simulink model "cpu2"  (R2020a)
settings: Solver=VariableStepAuto  StartTime=0.0  StopTime=10.0  RelTol=1e-3
libraries: simulink_extras x402, msbPllFoundation x1
(part 25 of 63)

== system cpu2/ALU/Multiplier/Subsystem2/Subsystem1/Subsystem1/Subsystem12 ==
  In1 : Inport
  In2 : Inport  Port=2
  Logical Operator1 : Logic  Operator=XOR  AllPortsSameDT=off  OutDataTypeStr=boolean
  Logical Operator2 : Logic  AllPortsSameDT=off  OutDataTypeStr=boolean
  Out1 : Outport
  Out2 : Outport  Port=2
  wires:
  In1/1 -> Logical Operator2/1, Logical Operator1/1
  Logical Operator1/1 -> Out1/1
  Logical Operator2/1 -> Out2/1
  In2/1 -> Logical Operator1/2, Logical Operator2/2

== system cpu2/ALU/Multiplier/Subsystem2/Subsystem1/Subsystem1/Subsystem13 ==
  In1 : Inport
  In2 : Inport  Port=2
  Logical Operator1 : Logic  Operator=XOR  AllPortsSameDT=off  OutDataTypeStr=boolean
  Logical Operator2 : Logic  AllPortsSameDT=off  OutDataTypeStr=boolean
  Out1 : Outport
  Out2 : Outport  Port=2
  wires:
  In1/1 -> Logical Operator2/1, Logical Operator1/1
  Logical Operator1/1 -> Out1/1
  Logical Operator2/1 -> Out2/1
  In2/1 -> Logical Operator1/2, Logical Operator2/2

== system cpu2/ALU/Multiplier/Subsystem2/Subsystem1/Subsystem1/Subsystem14 ==
  In1 : Inport
  In2 : Inport  Port=2
  Logical Operator1 : Logic  Operator=XOR  AllPortsSameDT=off  OutDataTypeStr=boolean
  Logical Operator2 : Logic  AllPortsSameDT=off  OutDataTypeStr=boolean
  Out1 : Outport
  Out2 : Outport  Port=2
  wires:
  In1/1 -> Logical Operator2/1, Logical Operator1/1
  Logical Operator1/1 -> Out1/1
  Logical Operator2/1 -> Out2/1
  In2/1 -> Logical Operator1/2, Logical Operator2/2

== system cpu2/ALU/Multiplier/Subsystem2/Subsystem1/Subsystem1/Subsystem2 ==
  In1 : Inport
  In2 : Inport  Port=2
  Logical Operator1 : Logic  Operator=XOR  AllPortsSameDT=off  OutDataTypeStr=boolean
  Logical Operator2 : Logic  AllPortsSameDT=off  OutDataTypeStr=boolean
  Out1 : Outport
  Out2 : Outport  Port=2
  wires:
  In1/1 -> Logical Operator2/1, Logical Operator1/1
  Logical Operator1/1 -> Out1/1
  Logical Operator2/1 -> Out2/1
  In2/1 -> Logical Operator1/2, Logical Operator2/2

== system cpu2/ALU/Multiplier/Subsystem2/Subsystem1/Subsystem1/Subsystem3 ==
  In1 : Inport
  In2 : Inport  Port=2
  In3 : Inport  Port=3
  Logical Operator : Logic  Operator=XOR  AllPortsSameDT=off  OutDataTypeStr=boolean
  Logical Operator1 : Logic  Operator=XOR  AllPortsSameDT=off  OutDataTypeStr=boolean
  Logical Operator2 : Logic  AllPortsSameDT=off  OutDataTypeStr=boolean
  Logical Operator3 : Logic  AllPortsSameDT=off  OutDataTypeStr=boolean
  Logical Operator4 : Logic  Operator=OR  AllPortsSameDT=off  OutDataTypeStr=boolean
  Out1 : Outport
  Out2 : Outport  Port=2
  wires:
  Logical Operator1/1 -> Out1/1
  Logical Operator2/1 -> Logical Operator4/1
  Logical Operator4/1 -> Out2/1
  In3/1 -> Logical Operator2/2, Logical Operator1/2
  In2/1 -> Logical Operator3/2, Logical Operator/2
  In1/1 -> Logical Operator3/1, Logical Operator/1
  Logical Operator3/1 -> Logical Operator4/2
  Logical Operator/1 -> Logical Operator2/1, Logical Operator1/1

== system cpu2/ALU/Multiplier/Subsystem2/Subsystem1/Subsystem1/Subsystem4 ==
  In1 : Inport
  In2 : Inport  Port=2
  In3 : Inport  Port=3
  Logical Operator : Logic  Operator=XOR  AllPortsSameDT=off  OutDataTypeStr=boolean
  Logical Operator1 : Logic  Operator=XOR  AllPortsSameDT=off  OutDataTypeStr=boolean
  Logical Operator2 : Logic  AllPortsSameDT=off  OutDataTypeStr=boolean
  Logical Operator3 : Logic  AllPortsSameDT=off  OutDataTypeStr=boolean
  Logical Operator4 : Logic  Operator=OR  AllPortsSameDT=off  OutDataTypeStr=boolean
  Out1 : Outport
  Out2 : Outport  Port=2
  wires:
  Logical Operator1/1 -> Out1/1
  Logical Operator2/1 -> Logical Operator4/1
  Logical Operator4/1 -> Out2/1
  In3/1 -> Logical Operator2/2, Logical Operator1/2
  In2/1 -> Logical Operator3/2, Logical Operator/2
  In1/1 -> Logical Operator3/1, Logical Operator/1
  Logical Operator3/1 -> Logical Operator4/2
  Logical Operator/1 -> Logical Operator2/1, Logical Operator1/1

== system cpu2/ALU/Multiplier/Subsystem2/Subsystem1/Subsystem1/Subsystem5 ==
  In1 : Inport
  In2 : Inport  Port=2
  Logical Operator1 : Logic  Operator=XOR  AllPortsSameDT=off  OutDataTypeStr=boolean
  Logical Operator2 : Logic  AllPortsSameDT=off  OutDataTypeStr=boolean
  Out1 : Outport
  Out2 : Outport  Port=2
  wires:
  In1/1 -> Logical Operator2/1, Logical Operator1/1
  Logical Operator1/1 -> Out1/1
  Logical Operator2/1 -> Out2/1
  In2/1 -> Logical Operator1/2, Logical Operator2/2

== system cpu2/ALU/Multiplier/Subsystem2/Subsystem1/Subsystem1/Subsystem6 ==
  In1 : Inport
  In2 : Inport  Port=2
  In3 : Inport  Port=3
  Logical Operator : Logic  Operator=XOR  AllPortsSameDT=off  OutDataTypeStr=boolean
  Logical Operator1 : Logic  Operator=XOR  AllPortsSameDT=off  OutDataTypeStr=boolean
  Logical Operator2 : Logic  AllPortsSameDT=off  OutDataTypeStr=boolean
  Logical Operator3 : Logic  AllPortsSameDT=off  OutDataTypeStr=boolean
  Logical Operator4 : Logic  Operator=OR  AllPortsSameDT=off  OutDataTypeStr=boolean
  Out1 : Outport
  Out2 : Outport  Port=2
  wires:
  Logical Operator1/1 -> Out1/1
  Logical Operator2/1 -> Logical Operator4/1
  Logical Operator4/1 -> Out2/1
  In3/1 -> Logical Operator2/2, Logical Operator1/2
  In2/1 -> Logical Operator3/2, Logical Operator/2
  In1/1 -> Logical Operator3/1, Logical Operator/1
  Logical Operator3/1 -> Logical Operator4/2
  Logical Operator/1 -> Logical Operator2/1, Logical Operator1/1

== system cpu2/ALU/Multiplier/Subsystem2/Subsystem1/Subsystem1/Subsystem7 ==
  In1 : Inport
  In2 : Inport  Port=2
  In3 : Inport  Port=3
  Logical Operator : Logic  Operator=XOR  AllPortsSameDT=off  OutDataTypeStr=boolean
  Logical Operator1 : Logic  Operator=XOR  AllPortsSameDT=off  OutDataTypeStr=boolean
  Logical Operator2 : Logic  AllPortsSameDT=off  OutDataTypeStr=boolean
  Logical Operator3 : Logic  AllPortsSameDT=off  OutDataTypeStr=boolean
  Logical Operator4 : Logic  Operator=OR  AllPortsSameDT=off  OutDataTypeStr=boolean
  Out1 : Outport
  Out2 : Outport  Port=2
  wires:
  Logical Operator1/1 -> Out1/1
  Logical Operator2/1 -> Logical Operator4/1
  Logical Operator4/1 -> Out2/1
  In3/1 -> Logical Operator2/2, Logical Operator1/2
  In2/1 -> Logical Operator3/2, Logical Operator/2
  In1/1 -> Logical Operator3/1, Logical Operator/1
  Logical Operator3/1 -> Logical Operator4/2
  Logical Operator/1 -> Logical Operator2/1, Logical Operator1/1

== system cpu2/ALU/Multiplier/Subsystem2/Subsystem1/Subsystem1/Subsystem8 ==
  In1 : Inport
  In2 : Inport  Port=2
  In3 : Inport  Port=3
  Logical Operator : Logic  Operator=XOR  AllPortsSameDT=off  OutDataTypeStr=boolean
  Logical Operator1 : Logic  Operator=XOR  AllPortsSameDT=off  OutDataTypeStr=boolean
  Logical Operator2 : Logic  AllPortsSameDT=off  OutDataTypeStr=boolean
  Logical Operator3 : Logic  AllPortsSameDT=off  OutDataTypeStr=boolean
  Logical Operator4 : Logic  Operator=OR  AllPortsSameDT=off  OutDataTypeStr=boolean
  Out1 : Outport
  Out2 : Outport  Port=2
  wires:
  Logical Operator1/1 -> Out1/1
  Logical Operator2/1 -> Logical Operator4/1
  Logical Operator4/1 -> Out2/1
  In3/1 -> Logical Operator2/2, Logical Operator1/2
  In2/1 -> Logical Operator3/2, Logical Operator/2
  In1/1 -> Logical Operator3/1, Logical Operator/1
  Logical Operator3/1 -> Logical Operator4/2
  Logical Operator/1 -> Logical Operator2/1, Logical Operator1/1

== system cpu2/ALU/Multiplier/Subsystem2/Subsystem1/Subsystem1/Subsystem9 ==
  In1 : Inport
  In2 : Inport  Port=2
  In3 : Inport  Port=3
  Logical Operator : Logic  Operator=XOR  AllPortsSameDT=off  OutDataTypeStr=boolean
  Logical Operator1 : Logic  Operator=XOR  AllPortsSameDT=off  OutDataTypeStr=boolean
  Logical Operator2 : Logic  AllPortsSameDT=off  OutDataTypeStr=boolean
  Logical Operator3 : Logic  AllPortsSameDT=off  OutDataTypeStr=boolean
  Logical Operator4 : Logic  Operator=OR  AllPortsSameDT=off  OutDataTypeStr=boolean
  Out1 : Outport
  Out2 : Outport  Port=2
  wires:
  Logical Operator1/1 -> Out1/1
  Logical Operator2/1 -> Logical Operator4/1
  Logical Operator4/1 -> Out2/1
  In3/1 -> Logical Operator2/2, Logical Operator1/2
  In2/1 -> Logical Operator3/2, Logical Operator/2
  In1/1 -> Logical Operator3/1, Logical Operator/1
  Logical Operator3/1 -> Logical Operator4/2
  Logical Operator/1 -> Logical Operator2/1, Logical Operator1/1

== system cpu2/ALU/Multiplier/Subsystem2/Subsystem1/Subsystem15/Subsystem ==
  In1 : Inport
  In2 : Inport  Port=2
  Logical Operator1 : Logic  Operator=XOR  AllPortsSameDT=off  OutDataTypeStr=boolean
  Logical Operator2 : Logic  AllPortsSameDT=off  OutDataTypeStr=boolean
  Out1 : Outport
  Out2 : Outport  Port=2
  wires:
  In1/1 -> Logical Operator2/1, Logical Operator1/1
  Logical Operator1/1 -> Out1/1
  Logical Operator2/1 -> Out2/1
  In2/1 -> Logical Operator1/2, Logical Operator2/2

== system cpu2/ALU/Multiplier/Subsystem2/Subsystem1/Subsystem15/Subsystem1 ==
  In1 : Inport
  In2 : Inport  Port=2
  In3 : Inport  Port=3
  Logical Operator : Logic  Operator=XOR  AllPortsSameDT=off  OutDataTypeStr=boolean
  Logical Operator1 : Logic  Operator=XOR  AllPortsSameDT=off  OutDataTypeStr=boolean
  Logical Operator2 : Logic  AllPortsSameDT=off  OutDataTypeStr=boolean
  Logical Operator3 : Logic  AllPortsSameDT=off  OutDataTypeStr=boolean
  Logical Operator4 : Logic  Operator=OR  AllPortsSameDT=off  OutDataTypeStr=boolean
  Out1 : Outport
  Out2 : Outport  Port=2
  wires:
  Logical Operator1/1 -> Out1/1
  Logical Operator2/1 -> Logical Operator4/1
  Logical Operator4/1 -> Out2/1
  In3/1 -> Logical Operator2/2, Logical Operator1/2
  In2/1 -> Logical Operator3/2, Logical Operator/2
  In1/1 -> Logical Operator3/1, Logical Operator/1
  Logical Operator3/1 -> Logical Operator4/2
  Logical Operator/1 -> Logical Operator2/1, Logical Operator1/1

== system cpu2/ALU/Multiplier/Subsystem2/Subsystem1/Subsystem15/Subsystem10 ==
  In1 : Inport
  In2 : Inport  Port=2
  Logical Operator1 : Logic  Operator=XOR  AllPortsSameDT=off  OutDataTypeStr=boolean
  Logical Operator2 : Logic  AllPortsSameDT=off  OutDataTypeStr=boolean
  Out1 : Outport
  Out2 : Outport  Port=2
  wires:
  In1/1 -> Logical Operator2/1, Logical Operator1/1
  Logical Operator1/1 -> Out1/1
  Logical Operator2/1 -> Out2/1
  In2/1 -> Logical Operator1/2, Logical Operator2/2

== system cpu2/ALU/Multiplier/Subsystem2/Subsystem1/Subsystem15/Subsystem11 ==
  In1 : Inport
  In2 : Inport  Port=2
  Logical Operator1 : Logic  Operator=XOR  AllPortsSameDT=off  OutDataTypeStr=boolean
  Logical Operator2 : Logic  AllPortsSameDT=off  OutDataTypeStr=boolean
  Out1 : Outport
  Out2 : Outport  Port=2
  wires:
  In1/1 -> Logical Operator2/1, Logical Operator1/1
  Logical Operator1/1 -> Out1/1
  Logical Operator2/1 -> Out2/1
  In2/1 -> Logical Operator1/2, Logical Operator2/2

== system cpu2/ALU/Multiplier/Subsystem2/Subsystem1/Subsystem15/Subsystem12 ==
  In1 : Inport
  In2 : Inport  Port=2
  Logical Operator1 : Logic  Operator=XOR  AllPortsSameDT=off  OutDataTypeStr=boolean
  Logical Operator2 : Logic  AllPortsSameDT=off  OutDataTypeStr=boolean
  Out1 : Outport
  Out2 : Outport  Port=2
  wires:
  In1/1 -> Logical Operator2/1, Logical Operator1/1
  Logical Operator1/1 -> Out1/1
  Logical Operator2/1 -> Out2/1
  In2/1 -> Logical Operator1/2, Logical Operator2/2

== system cpu2/ALU/Multiplier/Subsystem2/Subsystem1/Subsystem15/Subsystem13 ==
  In1 : Inport
  In2 : Inport  Port=2
  Logical Operator1 : Logic  Operator=XOR  AllPortsSameDT=off  OutDataTypeStr=boolean
  Logical Operator2 : Logic  AllPortsSameDT=off  OutDataTypeStr=boolean
  Out1 : Outport
  Out2 : Outport  Port=2
  wires:
  In1/1 -> Logical Operator2/1, Logical Operator1/1
  Logical Operator1/1 -> Out1/1
  Logical Operator2/1 -> Out2/1
  In2/1 -> Logical Operator1/2, Logical Operator2/2

== system cpu2/ALU/Multiplier/Subsystem2/Subsystem1/Subsystem15/Subsystem14 ==
  In1 : Inport
  In2 : Inport  Port=2
  Logical Operator1 : Logic  Operator=XOR  AllPortsSameDT=off  OutDataTypeStr=boolean
  Logical Operator2 : Logic  AllPortsSameDT=off  OutDataTypeStr=boolean
  Out1 : Outport
  Out2 : Outport  Port=2
  wires:
  In1/1 -> Logical Operator2/1, Logical Operator1/1
  Logical Operator1/1 -> Out1/1
  Logical Operator2/1 -> Out2/1
  In2/1 -> Logical Operator1/2, Logical Operator2/2

== system cpu2/ALU/Multiplier/Subsystem2/Subsystem1/Subsystem15/Subsystem2 ==
  In1 : Inport
  In2 : Inport  Port=2
  Logical Operator1 : Logic  Operator=XOR  AllPortsSameDT=off  OutDataTypeStr=boolean
  Logical Operator2 : Logic  AllPortsSameDT=off  OutDataTypeStr=boolean
  Out1 : Outport
  Out2 : Outport  Port=2
  wires:
  In1/1 -> Logical Operator2/1, Logical Operator1/1
  Logical Operator1/1 -> Out1/1
  Logical Operator2/1 -> Out2/1
  In2/1 -> Logical Operator1/2, Logical Operator2/2

== system cpu2/ALU/Multiplier/Subsystem2/Subsystem1/Subsystem15/Subsystem3 ==
  In1 : Inport
  In2 : Inport  Port=2
  In3 : Inport  Port=3
  Logical Operator : Logic  Operator=XOR  AllPortsSameDT=off  OutDataTypeStr=boolean
  Logical Operator1 : Logic  Operator=XOR  AllPortsSameDT=off  OutDataTypeStr=boolean
  Logical Operator2 : Logic  AllPortsSameDT=off  OutDataTypeStr=boolean
  Logical Operator3 : Logic  AllPortsSameDT=off  OutDataTypeStr=boolean
  Logical Operator4 : Logic  Operator=OR  AllPortsSameDT=off  OutDataTypeStr=boolean
  Out1 : Outport
  Out2 : Outport  Port=2
  wires:
  Logical Operator1/1 -> Out1/1
  Logical Operator2/1 -> Logical Operator4/1
  Logical Operator4/1 -> Out2/1
  In3/1 -> Logical Operator2/2, Logical Operator1/2
  In2/1 -> Logical Operator3/2, Logical Operator/2
  In1/1 -> Logical Operator3/1, Logical Operator/1
  Logical Operator3/1 -> Logical Operator4/2
  Logical Operator/1 -> Logical Operator2/1, Logical Operator1/1

== system cpu2/ALU/Multiplier/Subsystem2/Subsystem1/Subsystem15/Subsystem4 ==
  In1 : Inport
  In2 : Inport  Port=2
  In3 : Inport  Port=3
  Logical Operator : Logic  Operator=XOR  AllPortsSameDT=off  OutDataTypeStr=boolean
  Logical Operator1 : Logic  Operator=XOR  AllPortsSameDT=off  OutDataTypeStr=boolean
  Logical Operator2 : Logic  AllPortsSameDT=off  OutDataTypeStr=boolean
  Logical Operator3 : Logic  AllPortsSameDT=off  OutDataTypeStr=boolean
  Logical Operator4 : Logic  Operator=OR  AllPortsSameDT=off  OutDataTypeStr=boolean
  Out1 : Outport
  Out2 : Outport  Port=2
  wires:
  Logical Operator1/1 -> Out1/1
  Logical Operator2/1 -> Logical Operator4/1
  Logical Operator4/1 -> Out2/1
  In3/1 -> Logical Operator2/2, Logical Operator1/2
  In2/1 -> Logical Operator3/2, Logical Operator/2
  In1/1 -> Logical Operator3/1, Logical Operator/1
  Logical Operator3/1 -> Logical Operator4/2
  Logical Operator/1 -> Logical Operator2/1, Logical Operator1/1

== system cpu2/ALU/Multiplier/Subsystem2/Subsystem1/Subsystem15/Subsystem5 ==
  In1 : Inport
  In2 : Inport  Port=2
  Logical Operator1 : Logic  Operator=XOR  AllPortsSameDT=off  OutDataTypeStr=boolean
  Logical Operator2 : Logic  AllPortsSameDT=off  OutDataTypeStr=boolean
  Out1 : Outport
  Out2 : Outport  Port=2
  wires:
  In1/1 -> Logical Operator2/1, Logical Operator1/1
  Logical Operator1/1 -> Out1/1
  Logical Operator2/1 -> Out2/1
  In2/1 -> Logical Operator1/2, Logical Operator2/2

== system cpu2/ALU/Multiplier/Subsystem2/Subsystem1/Subsystem15/Subsystem6 ==
  In1 : Inport
  In2 : Inport  Port=2
  In3 : Inport  Port=3
  Logical Operator : Logic  Operator=XOR  AllPortsSameDT=off  OutDataTypeStr=boolean
  Logical Operator1 : Logic  Operator=XOR  AllPortsSameDT=off  OutDataTypeStr=boolean
  Logical Operator2 : Logic  AllPortsSameDT=off  OutDataTypeStr=boolean
  Logical Operator3 : Logic  AllPortsSameDT=off  OutDataTypeStr=boolean
  Logical Operator4 : Logic  Operator=OR  AllPortsSameDT=off  OutDataTypeStr=boolean
  Out1 : Outport
  Out2 : Outport  Port=2
  wires:
  Logical Operator1/1 -> Out1/1
  Logical Operator2/1 -> Logical Operator4/1
  Logical Operator4/1 -> Out2/1
  In3/1 -> Logical Operator2/2, Logical Operator1/2
  In2/1 -> Logical Operator3/2, Logical Operator/2
  In1/1 -> Logical Operator3/1, Logical Operator/1
  Logical Operator3/1 -> Logical Operator4/2
  Logical Operator/1 -> Logical Operator2/1, Logical Operator1/1

== system cpu2/ALU/Multiplier/Subsystem2/Subsystem1/Subsystem15/Subsystem7 ==
  In1 : Inport
  In2 : Inport  Port=2
  In3 : Inport  Port=3
  Logical Operator : Logic  Operator=XOR  AllPortsSameDT=off  OutDataTypeStr=boolean
  Logical Operator1 : Logic  Operator=XOR  AllPortsSameDT=off  OutDataTypeStr=boolean
  Logical Operator2 : Logic  AllPortsSameDT=off  OutDataTypeStr=boolean
  Logical Operator3 : Logic  AllPortsSameDT=off  OutDataTypeStr=boolean
  Logical Operator4 : Logic  Operator=OR  AllPortsSameDT=off  OutDataTypeStr=boolean
  Out1 : Outport
  Out2 : Outport  Port=2
  wires:
  Logical Operator1/1 -> Out1/1
  Logical Operator2/1 -> Logical Operator4/1
  Logical Operator4/1 -> Out2/1
  In3/1 -> Logical Operator2/2, Logical Operator1/2
  In2/1 -> Logical Operator3/2, Logical Operator/2
  In1/1 -> Logical Operator3/1, Logical Operator/1
  Logical Operator3/1 -> Logical Operator4/2
  Logical Operator/1 -> Logical Operator2/1, Logical Operator1/1

== system cpu2/ALU/Multiplier/Subsystem2/Subsystem1/Subsystem15/Subsystem8 ==
  In1 : Inport
  In2 : Inport  Port=2
  In3 : Inport  Port=3
  Logical Operator : Logic  Operator=XOR  AllPortsSameDT=off  OutDataTypeStr=boolean
  Logical Operator1 : Logic  Operator=XOR  AllPortsSameDT=off  OutDataTypeStr=boolean
  Logical Operator2 : Logic  AllPortsSameDT=off  OutDataTypeStr=boolean
  Logical Operator3 : Logic  AllPortsSameDT=off  OutDataTypeStr=boolean
  Logical Operator4 : Logic  Operator=OR  AllPortsSameDT=off  OutDataTypeStr=boolean
  Out1 : Outport
  Out2 : Outport  Port=2
  wires:
  Logical Operator1/1 -> Out1/1
  Logical Operator2/1 -> Logical Operator4/1
  Logical Operator4/1 -> Out2/1
  In3/1 -> Logical Operator2/2, Logical Operator1/2
  In2/1 -> Logical Operator3/2, Logical Operator/2
  In1/1 -> Logical Operator3/1, Logical Operator/1
  Logical Operator3/1 -> Logical Operator4/2
  Logical Operator/1 -> Logical Operator2/1, Logical Operator1/1

== system cpu2/ALU/Multiplier/Subsystem2/Subsystem1/Subsystem15/Subsystem9 ==
  In1 : Inport
  In2 : Inport  Port=2
  In3 : Inport  Port=3
  Logical Operator : Logic  Operator=XOR  AllPortsSameDT=off  OutDataTypeStr=boolean
  Logical Operator1 : Logic  Operator=XOR  AllPortsSameDT=off  OutDataTypeStr=boolean
  Logical Operator2 : Logic  AllPortsSameDT=off  OutDataTypeStr=boolean
  Logical Operator3 : Logic  AllPortsSameDT=off  OutDataTypeStr=boolean
  Logical Operator4 : Logic  Operator=OR  AllPortsSameDT=off  OutDataTypeStr=boolean
  Out1 : Outport
  Out2 : Outport  Port=2
  wires:
  Logical Operator1/1 -> Out1/1
  Logical Operator2/1 -> Logical Operator4/1
  Logical Operator4/1 -> Out2/1
  In3/1 -> Logical Operator2/2, Logical Operator1/2
  In2/1 -> Logical Operator3/2, Logical Operator/2
  In1/1 -> Logical Operator3/1, Logical Operator/1
  Logical Operator3/1 -> Logical Operator4/2
  Logical Operator/1 -> Logical Operator2/1, Logical Operator1/1

== system cpu2/ALU/Multiplier/Subsystem2/Subsystem1/Subsystem2/Subsystem ==
  In1 : Inport
  In2 : Inport  Port=2
  Logical Operator1 : Logic  Operator=XOR  AllPortsSameDT=off  OutDataTypeStr=boolean
  Logical Operator2 : Logic  AllPortsSameDT=off  OutDataTypeStr=boolean
  Out1 : Outport
  Out2 : Outport  Port=2
  wires:
  In1/1 -> Logical Operator2/1, Logical Operator1/1
  Logical Operator1/1 -> Out1/1
  Logical Operator2/1 -> Out2/1
  In2/1 -> Logical Operator1/2, Logical Operator2/2

== system cpu2/ALU/Multiplier/Subsystem2/Subsystem1/Subsystem2/Subsystem1 ==
  In1 : Inport
  In2 : Inport  Port=2
  In3 : Inport  Port=3
  Logical Operator : Logic  Operator=XOR  AllPortsSameDT=off  OutDataTypeStr=boolean
  Logical Operator1 : Logic  Operator=XOR  AllPortsSameDT=off  OutDataTypeStr=boolean
  Logical Operator2 : Logic  AllPortsSameDT=off  OutDataTypeStr=boolean
  Logical Operator3 : Logic  AllPortsSameDT=off  OutDataTypeStr=boolean
  Logical Operator4 : Logic  Operator=OR  AllPortsSameDT=off  OutDataTypeStr=boolean
  Out1 : Outport
  Out2 : Outport  Port=2
  wires:
  Logical Operator1/1 -> Out1/1
  Logical Operator2/1 -> Logical Operator4/1
  Logical Operator4/1 -> Out2/1
  In3/1 -> Logical Operator2/2, Logical Operator1/2
  In2/1 -> Logical Operator3/2, Logical Operator/2
  In1/1 -> Logical Operator3/1, Logical Operator/1
  Logical Operator3/1 -> Logical Operator4/2
  Logical Operator/1 -> Logical Operator2/1, Logical Operator1/1

== system cpu2/ALU/Multiplier/Subsystem2/Subsystem1/Subsystem2/Subsystem10 ==
  In1 : Inport
  In2 : Inport  Port=2
  Logical Operator1 : Logic  Operator=XOR  AllPortsSameDT=off  OutDataTypeStr=boolean
  Logical Operator2 : Logic  AllPortsSameDT=off  OutDataTypeStr=boolean
  Out1 : Outport
  Out2 : Outport  Port=2
  wires:
  In1/1 -> Logical Operator2/1, Logical Operator1/1
  Logical Operator1/1 -> Out1/1
  Logical Operator2/1 -> Out2/1
  In2/1 -> Logical Operator1/2, Logical Operator2/2

== system cpu2/ALU/Multiplier/Subsystem2/Subsystem1/Subsystem2/Subsystem11 ==
  In1 : Inport
  In2 : Inport  Port=2
  Logical Operator1 : Logic  Operator=XOR  AllPortsSameDT=off  OutDataTypeStr=boolean
  Logical Operator2 : Logic  AllPortsSameDT=off  OutDataTypeStr=boolean
  Out1 : Outport
  Out2 : Outport  Port=2
  wires:
  In1/1 -> Logical Operator2/1, Logical Operator1/1
  Logical Operator1/1 -> Out1/1
  Logical Operator2/1 -> Out2/1
  In2/1 -> Logical Operator1/2, Logical Operator2/2

== system cpu2/ALU/Multiplier/Subsystem2/Subsystem1/Subsystem2/Subsystem12 ==
  In1 : Inport
  In2 : Inport  Port=2
  Logical Operator1 : Logic  Operator=XOR  AllPortsSameDT=off  OutDataTypeStr=boolean
  Logical Operator2 : Logic  AllPortsSameDT=off  OutDataTypeStr=boolean
  Out1 : Outport
  Out2 : Outport  Port=2
  wires:
  In1/1 -> Logical Operator2/1, Logical Operator1/1
  Logical Operator1/1 -> Out1/1
  Logical Operator2/1 -> Out2/1
  In2/1 -> Logical Operator1/2, Logical Operator2/2

== system cpu2/ALU/Multiplier/Subsystem2/Subsystem1/Subsystem2/Subsystem13 ==
  In1 : Inport
  In2 : Inport  Port=2
  Logical Operator1 : Logic  Operator=XOR  AllPortsSameDT=off  OutDataTypeStr=boolean
  Logical Operator2 : Logic  AllPortsSameDT=off  OutDataTypeStr=boolean
  Out1 : Outport
  Out2 : Outport  Port=2
  wires:
  In1/1 -> Logical Operator2/1, Logical Operator1/1
  Logical Operator1/1 -> Out1/1
  Logical Operator2/1 -> Out2/1
  In2/1 -> Logical Operator1/2, Logical Operator2/2

== system cpu2/ALU/Multiplier/Subsystem2/Subsystem1/Subsystem2/Subsystem14 ==
  In1 : Inport
  In2 : Inport  Port=2
  Logical Operator1 : Logic  Operator=XOR  AllPortsSameDT=off  OutDataTypeStr=boolean
  Logical Operator2 : Logic  AllPortsSameDT=off  OutDataTypeStr=boolean
  Out1 : Outport
  Out2 : Outport  Port=2
  wires:
  In1/1 -> Logical Operator2/1, Logical Operator1/1
  Logical Operator1/1 -> Out1/1
  Logical Operator2/1 -> Out2/1
  In2/1 -> Logical Operator1/2, Logical Operator2/2

== system cpu2/ALU/Multiplier/Subsystem2/Subsystem1/Subsystem2/Subsystem2 ==
  In1 : Inport
  In2 : Inport  Port=2
  Logical Operator1 : Logic  Operator=XOR  AllPortsSameDT=off  OutDataTypeStr=boolean
  Logical Operator2 : Logic  AllPortsSameDT=off  OutDataTypeStr=boolean
  Out1 : Outport
  Out2 : Outport  Port=2
  wires:
  In1/1 -> Logical Operator2/1, Logical Operator1/1
  Logical Operator1/1 -> Out1/1
  Logical Operator2/1 -> Out2/1
  In2/1 -> Logical Operator1/2, Logical Operator2/2

== system cpu2/ALU/Multiplier/Subsystem2/Subsystem1/Subsystem2/Subsystem3 ==
  In1 : Inport
  In2 : Inport  Port=2
  In3 : Inport  Port=3
  Logical Operator : Logic  Operator=XOR  AllPortsSameDT=off  OutDataTypeStr=boolean
  Logical Operator1 : Logic  Operator=XOR  AllPortsSameDT=off  OutDataTypeStr=boolean
  Logical Operator2 : Logic  AllPortsSameDT=off  OutDataTypeStr=boolean
  Logical Operator3 : Logic  AllPortsSameDT=off  OutDataTypeStr=boolean
  Logical Operator4 : Logic  Operator=OR  AllPortsSameDT=off  OutDataTypeStr=boolean
  Out1 : Outport
  Out2 : Outport  Port=2
  wires:
  Logical Operator1/1 -> Out1/1
  Logical Operator2/1 -> Logical Operator4/1
  Logical Operator4/1 -> Out2/1
  In3/1 -> Logical Operator2/2, Logical Operator1/2
  In2/1 -> Logical Operator3/2, Logical Operator/2
  In1/1 -> Logical Operator3/1, Logical Operator/1
  Logical Operator3/1 -> Logical Operator4/2
  Logical Operator/1 -> Logical Operator2/1, Logical Operator1/1

== system cpu2/ALU/Multiplier/Subsystem2/Subsystem1/Subsystem2/Subsystem4 ==
  In1 : Inport
  In2 : Inport  Port=2
  In3 : Inport  Port=3
  Logical Operator : Logic  Operator=XOR  AllPortsSameDT=off  OutDataTypeStr=boolean
  Logical Operator1 : Logic  Operator=XOR  AllPortsSameDT=off  OutDataTypeStr=boolean
  Logical Operator2 : Logic  AllPortsSameDT=off  OutDataTypeStr=boolean
  Logical Operator3 : Logic  AllPortsSameDT=off  OutDataTypeStr=boolean
  Logical Operator4 : Logic  Operator=OR  AllPortsSameDT=off  OutDataTypeStr=boolean
  Out1 : Outport
  Out2 : Outport  Port=2
  wires:
  Logical Operator1/1 -> Out1/1
  Logical Operator2/1 -> Logical Operator4/1
  Logical Operator4/1 -> Out2/1
  In3/1 -> Logical Operator2/2, Logical Operator1/2
  In2/1 -> Logical Operator3/2, Logical Operator/2
  In1/1 -> Logical Operator3/1, Logical Operator/1
  Logical Operator3/1 -> Logical Operator4/2
  Logical Operator/1 -> Logical Operator2/1, Logical Operator1/1

== system cpu2/ALU/Multiplier/Subsystem2/Subsystem1/Subsystem2/Subsystem5 ==
  In1 : Inport
  In2 : Inport  Port=2
  Logical Operator1 : Logic  Operator=XOR  AllPortsSameDT=off  OutDataTypeStr=boolean
  Logical Operator2 : Logic  AllPortsSameDT=off  OutDataTypeStr=boolean
  Out1 : Outport
  Out2 : Outport  Port=2
  wires:
  In1/1 -> Logical Operator2/1, Logical Operator1/1
  Logical Operator1/1 -> Out1/1
  Logical Operator2/1 -> Out2/1
  In2/1 -> Logical Operator1/2, Logical Operator2/2

== system cpu2/ALU/Multiplier/Subsystem2/Subsystem1/Subsystem2/Subsystem6 ==
  In1 : Inport
  In2 : Inport  Port=2
  In3 : Inport  Port=3
  Logical Operator : Logic  Operator=XOR  AllPortsSameDT=off  OutDataTypeStr=boolean
  Logical Operator1 : Logic  Operator=XOR  AllPortsSameDT=off  OutDataTypeStr=boolean
  Logical Operator2 : Logic  AllPortsSameDT=off  OutDataTypeStr=boolean
  Logical Operator3 : Logic  AllPortsSameDT=off  OutDataTypeStr=boolean
  Logical Operator4 : Logic  Operator=OR  AllPortsSameDT=off  OutDataTypeStr=boolean
  Out1 : Outport
  Out2 : Outport  Port=2
  wires:
  Logical Operator1/1 -> Out1/1
  Logical Operator2/1 -> Logical Operator4/1
  Logical Operator4/1 -> Out2/1
  In3/1 -> Logical Operator2/2, Logical Operator1/2
  In2/1 -> Logical Operator3/2, Logical Operator/2
  In1/1 -> Logical Operator3/1, Logical Operator/1
  Logical Operator3/1 -> Logical Operator4/2
  Logical Operator/1 -> Logical Operator2/1, Logical Operator1/1

== system cpu2/ALU/Multiplier/Subsystem2/Subsystem1/Subsystem2/Subsystem7 ==
  In1 : Inport
  In2 : Inport  Port=2
  In3 : Inport  Port=3
  Logical Operator : Logic  Operator=XOR  AllPortsSameDT=off  OutDataTypeStr=boolean
  Logical Operator1 : Logic  Operator=XOR  AllPortsSameDT=off  OutDataTypeStr=boolean
  Logical Operator2 : Logic  AllPortsSameDT=off  OutDataTypeStr=boolean
  Logical Operator3 : Logic  AllPortsSameDT=off  OutDataTypeStr=boolean
  Logical Operator4 : Logic  Operator=OR  AllPortsSameDT=off  OutDataTypeStr=boolean
  Out1 : Outport
  Out2 : Outport  Port=2
  wires:
  Logical Operator1/1 -> Out1/1
  Logical Operator2/1 -> Logical Operator4/1
  Logical Operator4/1 -> Out2/1
  In3/1 -> Logical Operator2/2, Logical Operator1/2
  In2/1 -> Logical Operator3/2, Logical Operator/2
  In1/1 -> Logical Operator3/1, Logical Operator/1
  Logical Operator3/1 -> Logical Operator4/2
  Logical Operator/1 -> Logical Operator2/1, Logical Operator1/1

== system cpu2/ALU/Multiplier/Subsystem2/Subsystem1/Subsystem2/Subsystem8 ==
  In1 : Inport
  In2 : Inport  Port=2
  In3 : Inport  Port=3
  Logical Operator : Logic  Operator=XOR  AllPortsSameDT=off  OutDataTypeStr=boolean
  Logical Operator1 : Logic  Operator=XOR  AllPortsSameDT=off  OutDataTypeStr=boolean
  Logical Operator2 : Logic  AllPortsSameDT=off  OutDataTypeStr=boolean
  Logical Operator3 : Logic  AllPortsSameDT=off  OutDataTypeStr=boolean
  Logical Operator4 : Logic  Operator=OR  AllPortsSameDT=off  OutDataTypeStr=boolean
  Out1 : Outport
  Out2 : Outport  Port=2
  wires:
  Logical Operator1/1 -> Out1/1
  Logical Operator2/1 -> Logical Operator4/1
  Logical Operator4/1 -> Out2/1
  In3/1 -> Logical Operator2/2, Logical Operator1/2
  In2/1 -> Logical Operator3/2, Logical Operator/2
  In1/1 -> Logical Operator3/1, Logical Operator/1
  Logical Operator3/1 -> Logical Operator4/2
  Logical Operator/1 -> Logical Operator2/1, Logical Operator1/1

== system cpu2/ALU/Multiplier/Subsystem2/Subsystem1/Subsystem2/Subsystem9 ==
  In1 : Inport
  In2 : Inport  Port=2
  In3 : Inport  Port=3
  Logical Operator : Logic  Operator=XOR  AllPortsSameDT=off  OutDataTypeStr=boolean
  Logical Operator1 : Logic  Operator=XOR  AllPortsSameDT=off  OutDataTypeStr=boolean
  Logical Operator2 : Logic  AllPortsSameDT=off  OutDataTypeStr=boolean
  Logical Operator3 : Logic  AllPortsSameDT=off  OutDataTypeStr=boolean
  Logical Operator4 : Logic  Operator=OR  AllPortsSameDT=off  OutDataTypeStr=boolean
  Out1 : Outport
  Out2 : Outport  Port=2
  wires:
  Logical Operator1/1 -> Out1/1
  Logical Operator2/1 -> Logical Operator4/1
  Logical Operator4/1 -> Out2/1
  In3/1 -> Logical Operator2/2, Logical Operator1/2
  In2/1 -> Logical Operator3/2, Logical Operator/2
  In1/1 -> Logical Operator3/1, Logical Operator/1
  Logical Operator3/1 -> Logical Operator4/2
  Logical Operator/1 -> Logical Operator2/1, Logical Operator1/1

== system cpu2/ALU/Multiplier/Subsystem2/Subsystem1/Subsystem3/Subsystem ==
  In1 : Inport
  In2 : Inport  Port=2
  Logical Operator1 : Logic  Operator=XOR  AllPortsSameDT=off  OutDataTypeStr=boolean
  Logical Operator2 : Logic  AllPortsSameDT=off  OutDataTypeStr=boolean
  Out1 : Outport
  Out2 : Outport  Port=2
  wires:
  In1/1 -> Logical Operator2/1, Logical Operator1/1
  Logical Operator1/1 -> Out1/1
  Logical Operator2/1 -> Out2/1
  In2/1 -> Logical Operator1/2, Logical Operator2/2

== system cpu2/ALU/Multiplier/Subsystem2/Subsystem1/Subsystem3/Subsystem1 ==
  In1 : Inport
  In2 : Inport  Port=2
  In3 : Inport  Port=3
  Logical Operator : Logic  Operator=XOR  AllPortsSameDT=off  OutDataTypeStr=boolean
  Logical Operator1 : Logic  Operator=XOR  AllPortsSameDT=off  OutDataTypeStr=boolean
  Logical Operator2 : Logic  AllPortsSameDT=off  OutDataTypeStr=boolean
  Logical Operator3 : Logic  AllPortsSameDT=off  OutDataTypeStr=boolean
  Logical Operator4 : Logic  Operator=OR  AllPortsSameDT=off  OutDataTypeStr=boolean
  Out1 : Outport
  Out2 : Outport  Port=2
  wires:
  Logical Operator1/1 -> Out1/1
  Logical Operator2/1 -> Logical Operator4/1
  Logical Operator4/1 -> Out2/1
  In3/1 -> Logical Operator2/2, Logical Operator1/2
  In2/1 -> Logical Operator3/2, Logical Operator/2
  In1/1 -> Logical Operator3/1, Logical Operator/1
  Logical Operator3/1 -> Logical Operator4/2
  Logical Operator/1 -> Logical Operator2/1, Logical Operator1/1

== system cpu2/ALU/Multiplier/Subsystem2/Subsystem1/Subsystem3/Subsystem10 ==
  In1 : Inport
  In2 : Inport  Port=2
  Logical Operator1 : Logic  Operator=XOR  AllPortsSameDT=off  OutDataTypeStr=boolean
  Logical Operator2 : Logic  AllPortsSameDT=off  OutDataTypeStr=boolean
  Out1 : Outport
  Out2 : Outport  Port=2
  wires:
  In1/1 -> Logical Operator2/1, Logical Operator1/1
  Logical Operator1/1 -> Out1/1
  Logical Operator2/1 -> Out2/1
  In2/1 -> Logical Operator1/2, Logical Operator2/2

== system cpu2/ALU/Multiplier/Subsystem2/Subsystem1/Subsystem3/Subsystem11 ==
  In1 : Inport
  In2 : Inport  Port=2
  Logical Operator1 : Logic  Operator=XOR  AllPortsSameDT=off  OutDataTypeStr=boolean
  Logical Operator2 : Logic  AllPortsSameDT=off  OutDataTypeStr=boolean
  Out1 : Outport
  Out2 : Outport  Port=2
  wires:
  In1/1 -> Logical Operator2/1, Logical Operator1/1
  Logical Operator1/1 -> Out1/1
  Logical Operator2/1 -> Out2/1
  In2/1 -> Logical Operator1/2, Logical Operator2/2

== system cpu2/ALU/Multiplier/Subsystem2/Subsystem1/Subsystem3/Subsystem12 ==
  In1 : Inport
  In2 : Inport  Port=2
  Logical Operator1 : Logic  Operator=XOR  AllPortsSameDT=off  OutDataTypeStr=boolean
  Logical Operator2 : Logic  AllPortsSameDT=off  OutDataTypeStr=boolean
  Out1 : Outport
  Out2 : Outport  Port=2
  wires:
  In1/1 -> Logical Operator2/1, Logical Operator1/1
  Logical Operator1/1 -> Out1/1
  Logical Operator2/1 -> Out2/1
  In2/1 -> Logical Operator1/2, Logical Operator2/2

== system cpu2/ALU/Multiplier/Subsystem2/Subsystem1/Subsystem3/Subsystem13 ==
  In1 : Inport
  In2 : Inport  Port=2
  Logical Operator1 : Logic  Operator=XOR  AllPortsSameDT=off  OutDataTypeStr=boolean
  Logical Operator2 : Logic  AllPortsSameDT=off  OutDataTypeStr=boolean
  Out1 : Outport
  Out2 : Outport  Port=2
  wires:
  In1/1 -> Logical Operator2/1, Logical Operator1/1
  Logical Operator1/1 -> Out1/1
  Logical Operator2/1 -> Out2/1
  In2/1 -> Logical Operator1/2, Logical Operator2/2

== system cpu2/ALU/Multiplier/Subsystem2/Subsystem1/Subsystem3/Subsystem14 ==
  In1 : Inport
  In2 : Inport  Port=2
  Logical Operator1 : Logic  Operator=XOR  AllPortsSameDT=off  OutDataTypeStr=boolean
  Logical Operator2 : Logic  AllPortsSameDT=off  OutDataTypeStr=boolean
  Out1 : Outport
  Out2 : Outport  Port=2
  wires:
  In1/1 -> Logical Operator2/1, Logical Operator1/1
  Logical Operator1/1 -> Out1/1
  Logical Operator2/1 -> Out2/1
  In2/1 -> Logical Operator1/2, Logical Operator2/2

== system cpu2/ALU/Multiplier/Subsystem2/Subsystem1/Subsystem3/Subsystem2 ==
  In1 : Inport
  In2 : Inport  Port=2
  Logical Operator1 : Logic  Operator=XOR  AllPortsSameDT=off  OutDataTypeStr=boolean
  Logical Operator2 : Logic  AllPortsSameDT=off  OutDataTypeStr=boolean
  Out1 : Outport
  Out2 : Outport  Port=2
  wires:
  In1/1 -> Logical Operator2/1, Logical Operator1/1
  Logical Operator1/1 -> Out1/1
  Logical Operator2/1 -> Out2/1
  In2/1 -> Logical Operator1/2, Logical Operator2/2

== system cpu2/ALU/Multiplier/Subsystem2/Subsystem1/Subsystem3/Subsystem3 ==
  In1 : Inport
  In2 : Inport  Port=2
  In3 : Inport  Port=3
  Logical Operator : Logic  Operator=XOR  AllPortsSameDT=off  OutDataTypeStr=boolean
  Logical Operator1 : Logic  Operator=XOR  AllPortsSameDT=off  OutDataTypeStr=boolean
  Logical Operator2 : Logic  AllPortsSameDT=off  OutDataTypeStr=boolean
  Logical Operator3 : Logic  AllPortsSameDT=off  OutDataTypeStr=boolean
  Logical Operator4 : Logic  Operator=OR  AllPortsSameDT=off  OutDataTypeStr=boolean
  Out1 : Outport
  Out2 : Outport  Port=2
  wires:
  Logical Operator1/1 -> Out1/1
  Logical Operator2/1 -> Logical Operator4/1
  Logical Operator4/1 -> Out2/1
  In3/1 -> Logical Operator2/2, Logical Operator1/2
  In2/1 -> Logical Operator3/2, Logical Operator/2
  In1/1 -> Logical Operator3/1, Logical Operator/1
  Logical Operator3/1 -> Logical Operator4/2
  Logical Operator/1 -> Logical Operator2/1, Logical Operator1/1

== system cpu2/ALU/Multiplier/Subsystem2/Subsystem1/Subsystem3/Subsystem4 ==
  In1 : Inport
  In2 : Inport  Port=2
  In3 : Inport  Port=3
  Logical Operator : Logic  Operator=XOR  AllPortsSameDT=off  OutDataTypeStr=boolean
  Logical Operator1 : Logic  Operator=XOR  AllPortsSameDT=off  OutDataTypeStr=boolean
  Logical Operator2 : Logic  AllPortsSameDT=off  OutDataTypeStr=boolean
  Logical Operator3 : Logic  AllPortsSameDT=off  OutDataTypeStr=boolean
  Logical Operator4 : Logic  Operator=OR  AllPortsSameDT=off  OutDataTypeStr=boolean
  Out1 : Outport
  Out2 : Outport  Port=2
  wires:
  Logical Operator1/1 -> Out1/1
  Logical Operator2/1 -> Logical Operator4/1
  Logical Operator4/1 -> Out2/1
  In3/1 -> Logical Operator2/2, Logical Operator1/2
  In2/1 -> Logical Operator3/2, Logical Operator/2
  In1/1 -> Logical Operator3/1, Logical Operator/1
  Logical Operator3/1 -> Logical Operator4/2
  Logical Operator/1 -> Logical Operator2/1, Logical Operator1/1

== system cpu2/ALU/Multiplier/Subsystem2/Subsystem1/Subsystem3/Subsystem5 ==
  In1 : Inport
  In2 : Inport  Port=2
  Logical Operator1 : Logic  Operator=XOR  AllPortsSameDT=off  OutDataTypeStr=boolean
  Logical Operator2 : Logic  AllPortsSameDT=off  OutDataTypeStr=boolean
  Out1 : Outport
  Out2 : Outport  Port=2
  wires:
  In1/1 -> Logical Operator2/1, Logical Operator1/1
  Logical Operator1/1 -> Out1/1
  Logical Operator2/1 -> Out2/1
  In2/1 -> Logical Operator1/2, Logical Operator2/2

== system cpu2/ALU/Multiplier/Subsystem2/Subsystem1/Subsystem3/Subsystem6 ==
  In1 : Inport
  In2 : Inport  Port=2
  In3 : Inport  Port=3
  Logical Operator : Logic  Operator=XOR  AllPortsSameDT=off  OutDataTypeStr=boolean
  Logical Operator1 : Logic  Operator=XOR  AllPortsSameDT=off  OutDataTypeStr=boolean
  Logical Operator2 : Logic  AllPortsSameDT=off  OutDataTypeStr=boolean
  Logical Operator3 : Logic  AllPortsSameDT=off  OutDataTypeStr=boolean
  Logical Operator4 : Logic  Operator=OR  AllPortsSameDT=off  OutDataTypeStr=boolean
  Out1 : Outport
  Out2 : Outport  Port=2
  wires:
  Logical Operator1/1 -> Out1/1
  Logical Operator2/1 -> Logical Operator4/1
  Logical Operator4/1 -> Out2/1
  In3/1 -> Logical Operator2/2, Logical Operator1/2
  In2/1 -> Logical Operator3/2, Logical Operator/2
  In1/1 -> Logical Operator3/1, Logical Operator/1
  Logical Operator3/1 -> Logical Operator4/2
  Logical Operator/1 -> Logical Operator2/1, Logical Operator1/1

== system cpu2/ALU/Multiplier/Subsystem2/Subsystem1/Subsystem3/Subsystem7 ==
  In1 : Inport
  In2 : Inport  Port=2
  In3 : Inport  Port=3
  Logical Operator : Logic  Operator=XOR  AllPortsSameDT=off  OutDataTypeStr=boolean
  Logical Operator1 : Logic  Operator=XOR  AllPortsSameDT=off  OutDataTypeStr=boolean
  Logical Operator2 : Logic  AllPortsSameDT=off  OutDataTypeStr=boolean
  Logical Operator3 : Logic  AllPortsSameDT=off  OutDataTypeStr=boolean
  Logical Operator4 : Logic  Operator=OR  AllPortsSameDT=off  OutDataTypeStr=boolean
  Out1 : Outport
  Out2 : Outport  Port=2
  wires:
  Logical Operator1/1 -> Out1/1
  Logical Operator2/1 -> Logical Operator4/1
  Logical Operator4/1 -> Out2/1
  In3/1 -> Logical Operator2/2, Logical Operator1/2
  In2/1 -> Logical Operator3/2, Logical Operator/2
  In1/1 -> Logical Operator3/1, Logical Operator/1
  Logical Operator3/1 -> Logical Operator4/2
  Logical Operator/1 -> Logical Operator2/1, Logical Operator1/1

== system cpu2/ALU/Multiplier/Subsystem2/Subsystem1/Subsystem3/Subsystem8 ==
  In1 : Inport
  In2 : Inport  Port=2
  In3 : Inport  Port=3
  Logical Operator : Logic  Operator=XOR  AllPortsSameDT=off  OutDataTypeStr=boolean
  Logical Operator1 : Logic  Operator=XOR  AllPortsSameDT=off  OutDataTypeStr=boolean
  Logical Operator2 : Logic  AllPortsSameDT=off  OutDataTypeStr=boolean
  Logical Operator3 : Logic  AllPortsSameDT=off  OutDataTypeStr=boolean
  Logical Operator4 : Logic  Operator=OR  AllPortsSameDT=off  OutDataTypeStr=boolean
  Out1 : Outport
  Out2 : Outport  Port=2
  wires:
  Logical Operator1/1 -> Out1/1
  Logical Operator2/1 -> Logical Operator4/1
  Logical Operator4/1 -> Out2/1
  In3/1 -> Logical Operator2/2, Logical Operator1/2
  In2/1 -> Logical Operator3/2, Logical Operator/2
  In1/1 -> Logical Operator3/1, Logical Operator/1
  Logical Operator3/1 -> Logical Operator4/2
  Logical Operator/1 -> Logical Operator2/1, Logical Operator1/1

== system cpu2/ALU/Multiplier/Subsystem2/Subsystem1/Subsystem3/Subsystem9 ==
  In1 : Inport
  In2 : Inport  Port=2
  In3 : Inport  Port=3
  Logical Operator : Logic  Operator=XOR  AllPortsSameDT=off  OutDataTypeStr=boolean
  Logical Operator1 : Logic  Operator=XOR  AllPortsSameDT=off  OutDataTypeStr=boolean
  Logical Operator2 : Logic  AllPortsSameDT=off  OutDataTypeStr=boolean
  Logical Operator3 : Logic  AllPortsSameDT=off  OutDataTypeStr=boolean
  Logical Operator4 : Logic  Operator=OR  AllPortsSameDT=off  OutDataTypeStr=boolean
  Out1 : Outport
  Out2 : Outport  Port=2
  wires:
  Logical Operator1/1 -> Out1/1
  Logical Operator2/1 -> Logical Operator4/1
  Logical Operator4/1 -> Out2/1
  In3/1 -> Logical Operator2/2, Logical Operator1/2
  In2/1 -> Logical Operator3/2, Logical Operator/2
  In1/1 -> Logical Operator3/1, Logical Operator/1
  Logical Operator3/1 -> Logical Operator4/2
  Logical Operator/1 -> Logical Operator2/1, Logical Operator1/1

== system cpu2/ALU/Multiplier/Subsystem2/Subsystem1/Subsystem4/Subsystem ==
  In1 : Inport
  In2 : Inport  Port=2
  In3 : Inport  Port=3
  In4 : Inport  Port=4
  In5 : Inport  Port=5
  In6 : Inport  Port=6
  In7 : Inport  Port=7
  In8 : Inport  Port=8
  In9 : Inport  Port=9
  Logical Operator{,3,6,10} (4 alike) : Logic  AllPortsSameDT=off  OutDataTypeStr=boolean
  Logical Operator1 : Logic  Operator=OR  AllPortsSameDT=off  OutDataTypeStr=boolean
  Logical Operator11 : Logic  Operator=OR  Inputs=5  AllPortsSameDT=off  OutDataTypeStr=boolean
  Logical Operator12 : Logic  Inputs=4  AllPortsSameDT=off  OutDataTypeStr=boolean
  Logical Operator13 : Logic  Inputs=5  AllPortsSameDT=off  OutDataTypeStr=boolean
  Logical Operator2 : Logic  Inputs=3  AllPortsSameDT=off  OutDataTypeStr=boolean
  Logical Operator4 : Logic  Operator=OR  Inputs=3  AllPortsSameDT=off  OutDataTypeStr=boolean
  Logical Operator5 : Logic  Inputs=3  AllPortsSameDT=off  OutDataTypeStr=boolean
  Logical Operator7 : Logic  Operator=OR  Inputs=4  AllPortsSameDT=off  OutDataTypeStr=boolean
  Logical Operator8 : Logic  Inputs=4  AllPortsSameDT=off  OutDataTypeStr=boolean
  Logical Operator9 : Logic  Inputs=3  AllPortsSameDT=off  OutDataTypeStr=boolean
  Subsystem1 : Subsystem
  Subsystem2 : Subsystem
  Subsystem3 : Subsystem
  Subsystem4 : Subsystem
  Subsystem5 : Subsystem
  Subsystem6 : Subsystem
  Subsystem7 : Subsystem
  Subsystem8 : Subsystem
  Out1 : Outport
  Out2 : Outport  Port=2
  Out3 : Outport  Port=3
  Out4 : Outport  Port=4
  Out5 : Outport  Port=5
  wires:
  Logical Operator12/1 -> Logical Operator11/2
  Logical Operator9/1 -> Logical Operator11/3
  Logical Operator7/1 -> Subsystem7/3(In3)
  Logical Operator5/1 -> Logical Operator7/2
  Logical Operator13/1 -> Logical Operator11/1
  Logical Operator2/1 -> Logical Operator4/1
  Logical Operator/1 -> Logical Operator1/1
  Subsystem2/1(Out1) -> Out5/1
  Logical Operator3/1 -> Logical Operator4/2
  In3/1 -> Subsystem3/1(In1), Subsystem4/1(In1)
  Subsystem1/1(Out1) -> Logical Operator8/2, Logical Operator2/2, Logical Operator13/2, Logical Operator/1
  In5/1 -> Subsystem2/3(In3), Logical Operator13/1, Logical Operator8/1, Logical Operator2/1, Logical Operator/2
  Logical Operator4/1 -> Subsystem5/3(In3)
  Subsystem7/1(Out1) -> Out2/1
  Subsystem8/1(Out1) -> Logical Operator13/5, Logical Operator12/4, Logical Operator10/2, Logical Operator9/3
  Logical Operator11/1 -> Out1/1
  In9/1 -> Subsystem2/2(In2), Subsystem1/2(In2)
  In7/1 -> Subsystem5/2(In2), Subsystem6/2(In2)
  Logical Operator8/1 -> Logical Operator7/1
  Subsystem6/1(Out1) -> Logical Operator13/4, Logical Operator12/3, Logical Operator9/2, Logical Operator6/2, Logical Operator8/4, Logical Operator5/3
  In8/1 -> Subsystem3/2(In2), Subsystem4/2(In2)
  Subsystem5/1(Out1) -> Out3/1
  Subsystem1/2(Out2) -> Logical Operator12/1, Logical Operator3/1, Logical Operator1/2, Logical Operator5/1
  Subsystem4/1(Out1) -> Logical Operator8/3, Logical Operator5/2, Logical Operator3/2, Logical Operator2/3, Logical Operator13/3, Logical Operator12/2
  In1/1 -> Subsystem8/1(In1), Subsystem7/1(In1)
  Subsystem4/2(Out2) -> Logical Operator9/1, Logical Operator6/1, Logical Operator4/3
  Subsystem6/2(Out2) -> Logical Operator10/1, Logical Operator7/4
  Logical Operator10/1 -> Logical Operator11/4
  In2/1 -> Subsystem6/1(In1), Subsystem5/1(In1)
  In6/1 -> Subsystem7/2(In2), Subsystem8/2(In2)
  Logical Operator6/1 -> Logical Operator7/3
  In4/1 -> Subsystem2/1(In1), Subsystem1/1(In1)
  Subsystem8/2(Out2) -> Logical Operator11/5
  Subsystem3/1(Out1) -> Out4/1
  Logical Operator1/1 -> Subsystem3/3(In3)

== system cpu2/ALU/Multiplier/Subsystem2/Subsystem1/Subsystem4/Subsystem4 ==
  In1 : Inport
  In2 : Inport  Port=2
  In3 : Inport  Port=3
  In4 : Inport  Port=4
  In5 : Inport  Port=5
  In6 : Inport  Port=6
  In7 : Inport  Port=7
  In8 : Inport  Port=8
  In9 : Inport  Port=9
  Logical Operator{,3,6,10} (4 alike) : Logic  AllPortsSameDT=off  OutDataTypeStr=boolean
  Logical Operator1 : Logic  Operator=OR  AllPortsSameDT=off  OutDataTypeStr=boolean
  Logical Operator11 : Logic  Operator=OR  Inputs=5  AllPortsSameDT=off  OutDataTypeStr=boolean
  Logical Operator12 : Logic  Inputs=4  AllPortsSameDT=off  OutDataTypeStr=boolean
  Logical Operator13 : Logic  Inputs=5  AllPortsSameDT=off  OutDataTypeStr=boolean
  Logical Operator2 : Logic  Inputs=3  AllPortsSameDT=off  OutDataTypeStr=boolean
  Logical Operator4 : Logic  Operator=OR  Inputs=3  AllPortsSameDT=off  OutDataTypeStr=boolean
  Logical Operator5 : Logic  Inputs=3  AllPortsSameDT=off  OutDataTypeStr=boolean
  Logical Operator7 : Logic  Operator=OR  Inputs=4  AllPortsSameDT=off  OutDataTypeStr=boolean
  Logical Operator8 : Logic  Inputs=4  AllPortsSameDT=off  OutDataTypeStr=boolean
  Logical Operator9 : Logic  Inputs=3  AllPortsSameDT=off  OutDataTypeStr=boolean
  Subsystem1 : Subsystem
  Subsystem2 : Subsystem
  Subsystem3 : Subsystem
  Subsystem4 : Subsystem
  Subsystem5 : Subsystem
  Subsystem6 : Subsystem
  Subsystem7 : Subsystem
  Subsystem8 : Subsystem
  Out1 : Outport
  Out2 : Outport  Port=2
  Out3 : Outport  Port=3
  Out4 : Outport  Port=4
  Out5 : Outport  Port=5
  wires:
  Logical Operator12/1 -> Logical Operator11/2
  Logical Operator9/1 -> Logical Operator11/3
  Logical Operator7/1 -> Subsystem7/3(In3)
  Logical Operator5/1 -> Logical Operator7/2
  Logical Operator13/1 -> Logical Operator11/1
  Logical Operator2/1 -> Logical Operator4/1
  Logical Operator/1 -> Logical Operator1/1
  Subsystem2/1(Out1) -> Out5/1
  Logical Operator3/1 -> Logical Operator4/2
  In3/1 -> Subsystem3/1(In1), Subsystem4/1(In1)
  Subsystem1/1(Out1) -> Logical Operator8/2, Logical Operator2/2, Logical Operator13/2, Logical Operator/1
  In5/1 -> Subsystem2/3(In3), Logical Operator13/1, Logical Operator8/1, Logical Operator2/1, Logical Operator/2
  Logical Operator4/1 -> Subsystem5/3(In3)
  Subsystem7/1(Out1) -> Out2/1
  Subsystem8/1(Out1) -> Logical Operator13/5, Logical Operator12/4, Logical Operator10/2, Logical Operator9/3
  Logical Operator11/1 -> Out1/1
  In9/1 -> Subsystem2/2(In2), Subsystem1/2(In2)
  In7/1 -> Subsystem5/2(In2), Subsystem6/2(In2)
  Logical Operator8/1 -> Logical Operator7/1
  Subsystem6/1(Out1) -> Logical Operator13/4, Logical Operator12/3, Logical Operator9/2, Logical Operator6/2, Logical Operator8/4, Logical Operator5/3
  In8/1 -> Subsystem3/2(In2), Subsystem4/2(In2)
  Subsystem5/1(Out1) -> Out3/1
  Subsystem1/2(Out2) -> Logical Operator12/1, Logical Operator3/1, Logical Operator1/2, Logical Operator5/1
  Subsystem4/1(Out1) -> Logical Operator8/3, Logical Operator5/2, Logical Operator3/2, Logical Operator2/3, Logical Operator13/3, Logical Operator12/2
  In1/1 -> Subsystem8/1(In1), Subsystem7/1(In1)
  Subsystem4/2(Out2) -> Logical Operator9/1, Logical Operator6/1, Logical Operator4/3
  Subsystem6/2(Out2) -> Logical Operator10/1, Logical Operator7/4
  Logical Operator10/1 -> Logical Operator11/4
  In2/1 -> Subsystem6/1(In1), Subsystem5/1(In1)
  In6/1 -> Subsystem7/2(In2), Subsystem8/2(In2)
  Logical Operator6/1 -> Logical Operator7/3
  In4/1 -> Subsystem2/1(In1), Subsystem1/1(In1)
  Subsystem8/2(Out2) -> Logical Operator11/5
  Subsystem3/1(Out1) -> Out4/1
  Logical Operator1/1 -> Subsystem3/3(In3)
